simulink model "ad_fbl_ctrl"  (R2021a)
settings: Solver=VariableStepAuto  StartTime=0.0  StopTime=tf  FixedStep=0.002  RelTol=1e-3
values from neighbouring files (symbols this model uses):
  apply_noise = 1    [fbl.m]
  noise_a = -20e-7    (= -2e-06)    [main.m]
  noise_b = -50e-7    (= -5e-06)    [main.m]
  r = 0    [main.m]
  Ts = 0.02    [main.m]
  x0 = [950; 550; 6e-4]    [main.m]
  x10 = 1000    [main.m]
  x20 = 550    [main.m]
undefined symbols (not defined in the file or in its folder): DiscIntNeverNeededParam, error_thresh, gain_locking, k_apt, ke_apt, kf_apt
libraries: simulink x3
settings Model: Creator=micma  LastModifiedBy=micma

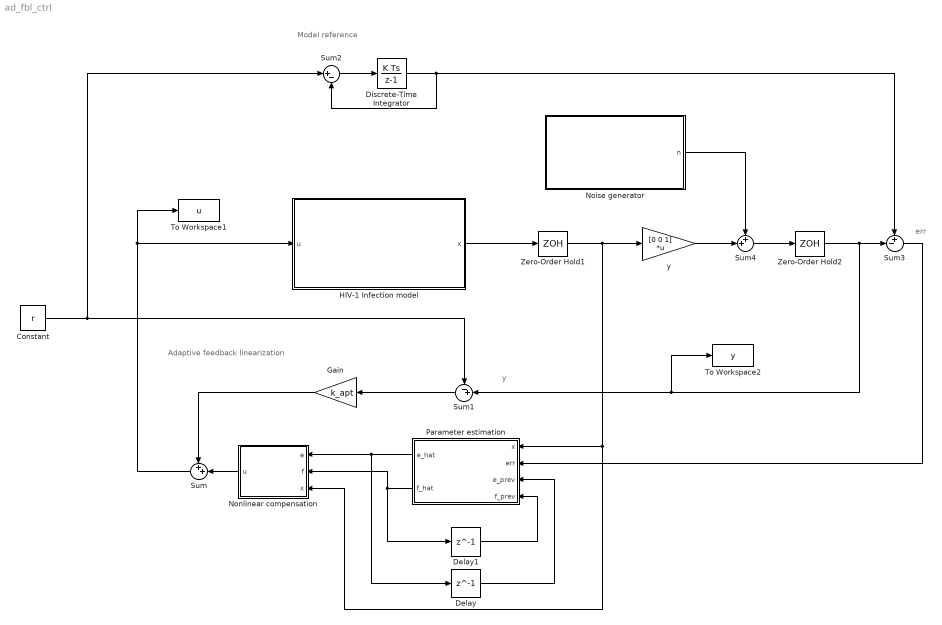
== system ad_fbl_ctrl ==
  note: y
  note: Model reference
  note: err
  note: Adaptive feedback linearization
  Constant : Constant  Value=r
  Delay : Delay  DelayLength=1  InitialCondition=0
  Delay1 : Delay  DelayLength=1  InitialCondition=0
  Discrete-Time Integrator : DiscreteIntegrator  gainval=k_apt  SampleTime=Ts  ICPrevOutput=DiscIntNeverNeededParam  ICPrevScaledInput=DiscIntNeverNeededParam
  Gain : Gain  Gain=k_apt
  HIV-1 Infection model : Subsystem
  Noise generator : Subsystem
  Nonlinear compensation : Subsystem
  Parameter estimation : Subsystem
  Sum : Sum  Inputs=++|
  Sum1 : Sum  Inputs=-+|
  Sum2 : Sum  Inputs=|+-
  Sum3 : Sum  Inputs=+-|
  Sum4 : Sum  Inputs=++|
  To Workspace1 : ToWorkspace  VariableName=u  SaveFormat=Timeseries  SampleTime=-1
  To Workspace2 : ToWorkspace  VariableName=y  SaveFormat=Timeseries  SampleTime=-1
  Zero-Order Hold1 : ZeroOrderHold  SampleTime=Ts
  Zero-Order Hold2 : ZeroOrderHold  SampleTime=Ts
  y : Gain  Gain=[0 0 1]  Multiplication=Matrix(K*u)
  wires:
  Zero-Order Hold1/1 -> Nonlinear compensation/3(x), Parameter estimation/1(x), y/1
  HIV-1 Infection model/1(x) -> Zero-Order Hold1/1
  Sum/1 -> To Workspace1/1, HIV-1 Infection model/1(u)
  Sum1/1 -> Gain/1
  Parameter estimation/2(f_hat) -> Nonlinear compensation/2(f), Delay1/1
  Parameter estimation/1(e_hat) -> Nonlinear compensation/1(e), Delay/1
  Delay/1 -> Parameter estimation/3(e_prev)
  Delay1/1 -> Parameter estimation/4(f_prev)
  Gain/1 -> Sum/1
  Nonlinear compensation/1(u) -> Sum/2
  Constant/1 -> Sum2/1, Sum1/1
  Sum2/1 -> Discrete-Time Integrator/1
  Discrete-Time Integrator/1 -> Sum3/1, Sum2/2
  Sum3/1 -> Parameter estimation/2(err)
  Noise generator/1(n) -> Sum4/1
  y/1 -> Sum4/2
  Zero-Order Hold2/1 -> Sum3/2, To Workspace2/1, Sum1/2
  Sum4/1 -> Zero-Order Hold2/1

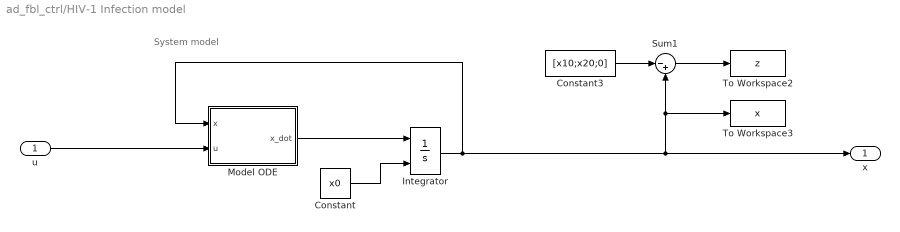
== system ad_fbl_ctrl/HIV-1 Infection model ==
  note: System model
  u : Inport
  Constant : Constant  Value=x0
  Constant3 : Constant  Value=[x10;x20;0]
  Integrator : Integrator  InitialConditionSource=external
  Model ODE : MATLAB Function  TreatAsAtomicUnit=on
  Sum1 : Sum  Inputs=|-+
  To Workspace2 : ToWorkspace  VariableName=z  SaveFormat=Timeseries  SampleTime=-1
  To Workspace3 : ToWorkspace  VariableName=x  SaveFormat=Timeseries  SampleTime=-1
  x : Outport
  wires:
  Model ODE/1(x_dot) -> Integrator/1
  Constant/1 -> Integrator/2
  Integrator/1 -> x/1, To Workspace3/1, Sum1/2, Model ODE/1(x)
  u/1 -> Model ODE/2(u)
  Constant3/1 -> Sum1/1
  Sum1/1 -> To Workspace2/1

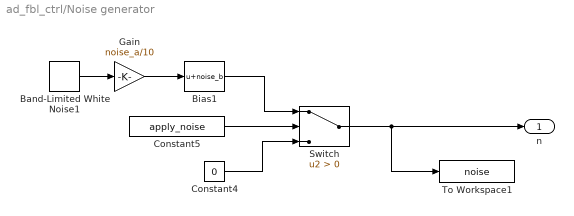
== system ad_fbl_ctrl/Noise generator ==
  Band-Limited White Noise1 : simulink/Sources/Band-Limited White Noise  Cov=[.1]  Ts=Ts*0.1  seed=[23341]
  Bias1 : Bias  Bias=noise_b
  Constant4 : Constant  Value=0
  Constant5 : Constant  Value=apply_noise
  Gain : Gain  Gain=noise_a/10
  Switch : Switch  Criteria=u2 > Threshold
  To Workspace1 : ToWorkspace  VariableName=noise  SaveFormat=Timeseries  SampleTime=-1
  n : Outport
  wires:
  Constant5/1 -> Switch/2
  Constant4/1 -> Switch/3
  Switch/1 -> n/1, To Workspace1/1
  Bias1/1 -> Switch/1
  Band-Limited White Noise1/1 -> Gain/1
  Gain/1 -> Bias1/1

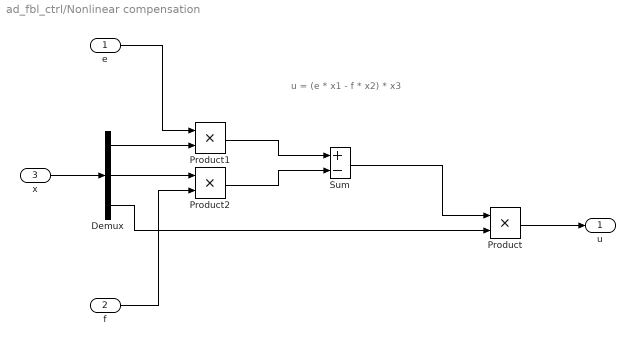
== system ad_fbl_ctrl/Nonlinear compensation ==
  note: u = (e * x1 - f * x2) * x3
  e : Inport
  f : Inport  Port=2
  x : Inport  Port=3
  Demux : Demux  Outputs=3
  Product : Product
  Product1 : Product
  Product2 : Product
  Sum : Sum  Inputs=+-
  u : Outport
  wires:
  x/1 -> Demux/1
  Demux/1 -> Product1/2
  Demux/2 -> Product2/1
  Product1/1 -> Sum/1
  Product2/1 -> Sum/2
  Sum/1 -> Product/1
  Demux/3 -> Product/2
  Product/1 -> u/1
  e/1 -> Product1/1
  f/1 -> Product2/2

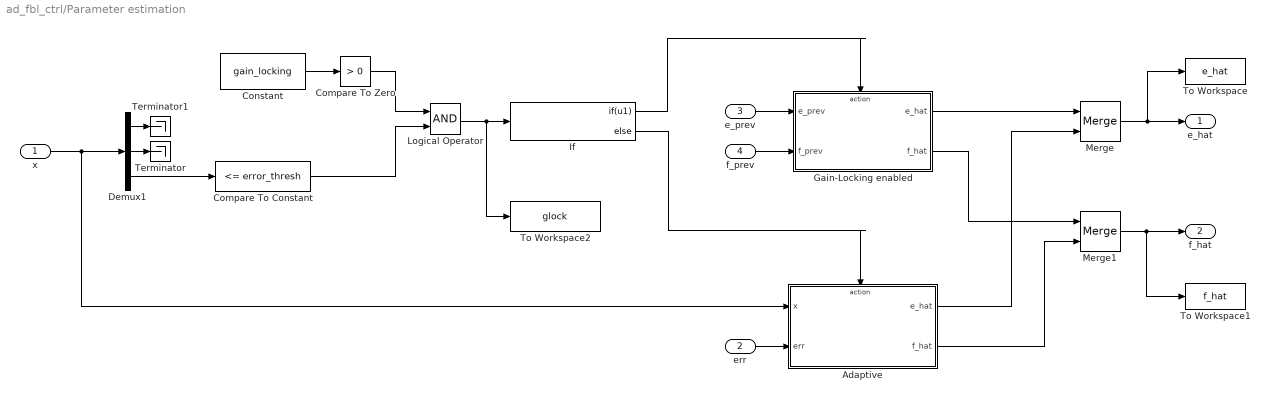
== system ad_fbl_ctrl/Parameter estimation ==
  x : Inport
  err : Inport  Port=2
  e_prev : Inport  Port=3
  f_prev : Inport  Port=4
  Adaptive : Subsystem  TreatAsAtomicUnit=on
  Compare To Constant : simulink/Logic and Bit Operations/Compare To Constant  relop=<=  const=error_thresh  OutDataTypeStr=boolean  ZeroCross=off
  Compare To Zero : simulink/Logic and Bit Operations/Compare To Zero  relop=>  OutDataTypeStr=boolean
  Constant : Constant  Value=gain_locking
  Demux1 : Demux  Outputs=3
  Gain-Locking enabled : Subsystem  TreatAsAtomicUnit=on
  If : If  IfExpression=u1
  Logical Operator : Logic  AllPortsSameDT=off  OutDataTypeStr=boolean
  Merge : Merge  InitialOutput=0
  Merge1 : Merge  InitialOutput=0
  Terminator : Terminator
  Terminator1 : Terminator
  To Workspace : ToWorkspace  VariableName=e_hat  SaveFormat=Timeseries  SampleTime=-1
  To Workspace1 : ToWorkspace  VariableName=f_hat  SaveFormat=Timeseries  SampleTime=-1
  To Workspace2 : ToWorkspace  VariableName=glock  SaveFormat=Timeseries  SampleTime=-1
  e_hat : Outport
  f_hat : Outport  Port=2
  wires:
  Compare To Constant/1 -> Logical Operator/2
  Gain-Locking enabled/1(e_hat) -> Merge/1
  Adaptive/1(e_hat) -> Merge/2
  Gain-Locking enabled/2(f_hat) -> Merge1/1
  Adaptive/2(f_hat) -> Merge1/2
  If/2 -> Adaptive/Action
  Constant/1 -> Compare To Zero/1
  Logical Operator/1 -> If/1, To Workspace2/1
  Compare To Zero/1 -> Logical Operator/1
  Demux1/3 -> Compare To Constant/1
  If/1 -> Gain-Locking enabled/Action
  x/1 -> Demux1/1, Adaptive/1(x)
  Demux1/2 -> Terminator/1
  Demux1/1 -> Terminator1/1
  e_prev/1 -> Gain-Locking enabled/1(e_prev)
  f_prev/1 -> Gain-Locking enabled/2(f_prev)
  Merge/1 -> To Workspace/1, e_hat/1
  Merge1/1 -> To Workspace1/1, f_hat/1
  err/1 -> Adaptive/2(err)

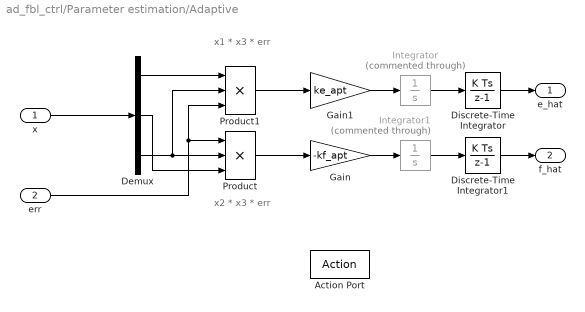
== system ad_fbl_ctrl/Parameter estimation/Adaptive ==
  note: x2 * x3 * err
  note: x1 * x3 * err
  x : Inport
  err : Inport  Port=2
  Action Port : ActionPort  ActionPortLabel=else
  Demux : Demux  Outputs=3
  Discrete-Time Integrator : DiscreteIntegrator  SampleTime=-1  ICPrevOutput=DiscIntNeverNeededParam  ICPrevScaledInput=DiscIntNeverNeededParam
  Discrete-Time Integrator1 : DiscreteIntegrator  SampleTime=-1  ICPrevOutput=DiscIntNeverNeededParam  ICPrevScaledInput=DiscIntNeverNeededParam
  Gain : Gain  Gain=-kf_apt
  Gain1 : Gain  Gain=ke_apt
  Integrator : Integrator  Commented=through
  Integrator1 : Integrator  Commented=through
  Product : Product  Inputs=3
  Product1 : Product  Inputs=3
  e_hat : Outport
  f_hat : Outport  Port=2
  wires:
  x/1 -> Demux/1
  Product1/1 -> Gain1/1
  Product/1 -> Gain/1
  Gain1/1 -> Integrator/1
  Integrator/1 -> Discrete-Time Integrator/1
  Gain/1 -> Integrator1/1
  Integrator1/1 -> Discrete-Time Integrator1/1
  Discrete-Time Integrator/1 -> e_hat/1
  Discrete-Time Integrator1/1 -> f_hat/1
  Demux/1 -> Product1/1
  Demux/3 -> Product/2, Product1/2
  err/1 -> Product/1, Product1/3
  Demux/2 -> Product/3

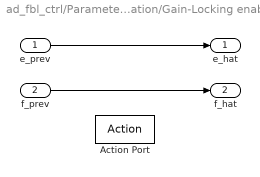
== system ad_fbl_ctrl/Parameter estimation/Gain-Locking enabled ==
  e_prev : Inport
  f_prev : Inport  Port=2
  Action Port : ActionPort  ActionPortLabel=if(u1)
  e_hat : Outport
  f_hat : Outport  Port=2
  wires:
  f_prev/1 -> f_hat/1
  e_prev/1 -> e_hat/1

== matlab function ad_fbl_ctrl/HIV-1 Infection model/Model ODE ==
  data: x input; u input; x_dot output; params parameter
function x_dot = ode(x, u, params)
x_dot = modelODE(x, u, params);
end
